simulink model "A3"  (R2024a)
settings: Solver=VariableStepAuto  StartTime=0.0  StopTime=10.0  RelTol=1e-3
settings Model: Creator=Flipper  LastModifiedBy=Flipper

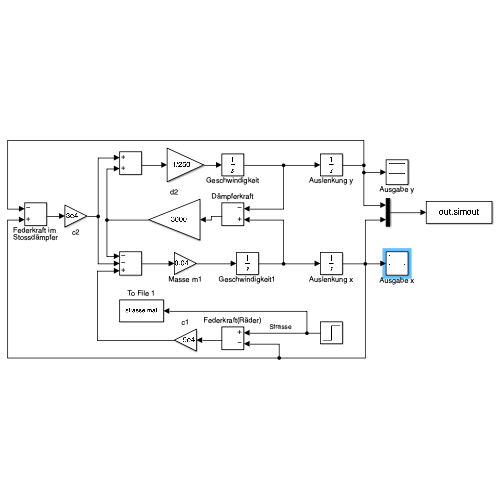
[thumbnail: Simulink's stored preview of the top-level diagram]
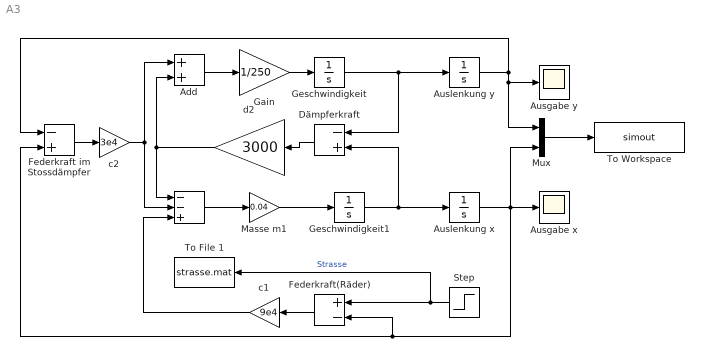
== system A3 ==
  " " : Sum  Inputs=--+
  Add : Sum
  Ausgabe x : Scope
  Ausgabe y : Scope
  Auslenkung x : Integrator
  Auslenkung y : Integrator
  Dämpferkraft : Sum  Inputs=-+
  Federkraft im Stossdämpfer : Sum  Inputs=-+
  Federkraft(Räder) : Sum  Inputs=+-
  Gain : Gain  Gain=1/250
  Geschwindigkeit : Integrator
  Geschwindigkeit1 : Integrator
  Masse m1 : Gain  Gain=0.04
  Mux : Mux  Inputs=2
  Step : Step  Time=0  SampleTime=0
  To File 1 : ToFile  Filename=strasse.mat  SaveFormat=Timeseries
  To Workspace : ToWorkspace  VariableName=simout  SaveFormat=Timeseries  SampleTime=-1
  c1 : Gain  Gain=9e4
  c2 : Gain  Gain=3e4
  d2 : Gain  Gain=3000
  wires:
  Dämpferkraft/1 -> d2/1
  Add/1 -> Gain/1
  Gain/1 -> Geschwindigkeit/1
  Geschwindigkeit/1 -> Dämpferkraft/1, Auslenkung y/1
  Auslenkung y/1 -> Mux/1, Ausgabe y/1, Federkraft im Stossdämpfer/1
  Federkraft im Stossdämpfer/1 -> c2/1
  c2/1 -> " "/2, Add/1
  d2/1 -> Add/2, " "/1
  Mux/1 -> To Workspace/1
  Auslenkung x/1 -> Federkraft im Stossdämpfer/2, Federkraft(Räder)/2, Ausgabe x/1, Mux/2
  Geschwindigkeit1/1 -> Auslenkung x/1, Dämpferkraft/2
  Masse m1/1 -> Geschwindigkeit1/1
  " "/1 -> Masse m1/1
  Step/1 -> To File 1/1, Federkraft(Räder)/1  "Strasse"
  Federkraft(Räder)/1 -> c1/1
  c1/1 -> " "/3
